simulink model "Backhoe_Arm"  (R2020a)
settings: Solver=ode23t  StartTime=0.0  StopTime=60  RelTol=1e-3  EnableMultiTasking=on
PostLoadFcn:
  | warning off simscape:compiler:sli:init:SolverNotRecommended
  | 
  | warning off sm:sli:visualization:UnsupportedSimMode
  | warning off sm:sli:setup:compile:LocalSolverNotSupported
  | warning off sm:compiler:state:UnsatisfiedDesiredTarget
  | 
  | warning off xPCTarget:sampleTime:sampleTimeInvariance
  | warning off Simulink:blocks:MatchingFromNotFound
model workspace (MAT data in the model file):
  cylinderGray = [0.6 0.6 0.6]
  darkOrange = [0.8 0.5 0]
  glassBlue = [0.2 0.2 1]
  gray = [0.3 0.3 0.3]
  orange = [0.8 0.65 0]
  pistonGray = [0.4 0.4 0.4]
  rhoGlass = 2500
  rhoRubber = 1500
  rhoSteel = 7800
  tireBlack = [0.1 0.1 0.1]
  wheelGray = [0.6 0.6 0.6]
  yellow = [0.8 0.8 0]
undefined symbols (not defined in the file or in its folder): BH_Param, sigbuilder_block, X, Y, Z
libraries: sm_lib x98, fl_lib x31, Backhoe_Lib x28, nesl_utility x22, sh_lib x9, slrtlib x1
(part 1 of 4)
CloseFcn:
  | try,close(h1_Backhoe_Arm),end
  | clear h1_Backhoe_Arm
  | try,close(h2_Backhoe_Arm),end
  | clear h2_Backhoe_Arm
  | 
  | clear simlog_Backhoe_Arm
  | clear logsout_Backhoe_Arm
Description:
  | Backhoe Arm
  | 
  | Copyright 2014-2020 The MathWorks, Inc.
settings Model: ExtModeTrigDuration=2500  Creator=smiller  LastModifiedBy=smiller
settings DataIOCC: MaxDataPoints=10000  SaveFormat=Array  ReturnWorkspaceOutputs=off  SignalLoggingName=logsout_Backhoe_Arm
settings OptimizationCC: BlockReduction=off  OptimizeBlockIOStorage=off  BufferReuse=off  GlobalBufferReuse=off  ExpressionFolding=off  ExpressionDepthLimit=2147483647  LocalBlockOutputs=off  LifeSpan=inf  OptimizeDataStoreBuffers=off  BusAssignmentInplaceUpdate=off
settings DebuggingCC: UnderspecifiedInitializationDetection=Classic  MergeDetectMultiDrivingBlocksExec=none  MultiTaskDSMMsg=warning  MultiTaskCondExecSysMsg=none  AllowSymbolicDim=off  StateNameClashWarn=warning  PregeneratedLibrarySubsystemCodeDiagnostic=none  SFUnexpectedBacktrackingDiag=warning  SFNoUnconditionalDefaultTransitionDiag=warning  SFExecutionAtInitializationDiag=none  ArithmeticOperatorsInVariantConditions=warning
settings HardwareCC: ProdBitPerPointer=32  ProdBitPerSizeT=32  ProdBitPerPtrDiffT=32  ProdLargestAtomicFloat=None  ProdWordSize=32  ProdLongLongMode=on  ProdHWDeviceType=Generic->32-bit x86 compatible
settings ModelReferenceCC: PropagateSignalLabelsOutOfModel=off
settings SFSimCC: SimUseLocalCustomCode=off  CustomCodeUndefinedFunction=UseInterfaceOnly
settings RTWCC: Description=Simulink Real-Time  SystemTargetFile=slrt.tlc  TemplateMakefile=slrt_default_tmf  RTWUseLocalCustomCode=off  CodeExecutionProfiling=on  RTWCompilerOptimization=on
settings CodeAppCC: StateflowObjectComments=on
settings SimulinkRealTimeCC: RL32LogBufSizeModifier=300000
settings ConfigComp: CovMetricSettings=dw  CovHtmlReporting=on  CovSaveCumulativeToWorkspaceVar=on  CovSaveSingleToWorkspaceVar=on  CovExternalEMLEnable=off  CovSFcnEnable=off
settings SimscapeCC: ExplicitSolverDiagnosticOptions=none  SimscapeNormalizeSystem=off  SimscapeLogType=all  SimscapeLogSimulationStatistics=on  SimscapeLogName=simlog_Backhoe_Arm  SimscapeLogDataHistory=150000
settings ConfigurationSet: Description=SimMechanics 2G
settings ExplorerConfigSet: InternalSimMechanicsExplorerSettings="<ExplorerConfiguration><canonicalview>default</canonicalview><AnimationSetting><BasePlaybackSpeed>1.0</BasePlaybackSpeed><PlaybackSpeedFactor>1.0</PlaybackSpeedFactor></AnimationSetting><TilePanel><TileInfo><Tiles Columns=\"1\" Count=\"1\" Rows=\"1\"><Column Weight=\"1\"/><Row Weight=\"1\"/><Tile Height=\"1\" Width=\"1\" X=\"0\" Y=\"0\"/></Tiles></TileInfo><SceneInfo><SceneViewer><BGColor><R>1</R><G>1</G><B>1</B></BGColor><Camera><DoPerspective>off</DoPerspective><Position><X>16.2117166228468328</X><Y>-13.0612993780048647</Y><Z>8.35403361976682568</Z></Position><Center><X>-0.886183199059584648</X><Y>-6.57974503836197222</Y><Z>3.30771103067373451</Z></Center><Up><X>-0.262324217563679185</X><Y>0.057951672533943753</Y><Z>0.963238085070416306</Z></Up><ViewLimDist>1</ViewLimDist><YLim>5.09128224849700928</YLim><XLim>8.0878249386863228</XLim></Camera></SceneViewer></SceneInfo></TilePanel><MechEditorPanel><Cameras/><GfxPanelCameraMap/><VideoCreator><PlaybackSpeedRatio>1.0</PlaybackSpeedRatio><FrameRate>30</FrameRate><VideoFormat>Motion JPEG AVI</VideoFormat><FrameSize>auto</FrameSize></VideoCreator></MechEditorPanel></ExplorerConfiguration>"

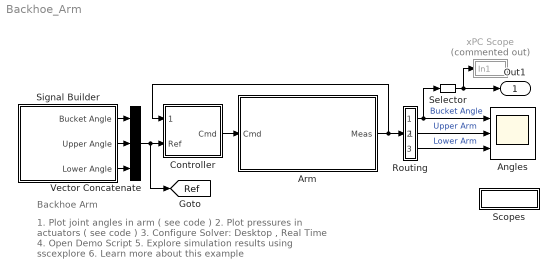
== system Backhoe_Arm ==
  note: 1. Plot joint angles in arm ( see code )
      | 2. Plot pressures in actuators ( see code )
      | 3. Configure Solver: Desktop , Real Time
      | 4. Open Demo Script
      | 5. Explore simulation results using sscexplore
      | 6. Learn more about this example
  note: Backhoe Arm
  Angles : Scope  NumInputPorts=3
  Arm : Subsystem  Tag=PublishSubsystem
      mask Display:
      | image('Backhoe_Arm_IMAGE.jpg');
      | port_label('input',1,'Cmd');
      | port_label('Output',1,'Meas');
  Controller : Subsystem
  Routing : Subsystem
  Scopes : Subsystem
  Selector : Selector  InputPortWidth=2  IndexOptions=Index vector (dialog)  Indices=[1]  OutputSizes=1
  Signal Builder : Subsystem  Tag=STV Subsys  LoadFcn=sigbuilder_block('load');  StartFcn=sigbuilder_block('start');  StopFcn=sigbuilder_block('stop');  ClipboardFcn=sigbuilder_block('clipboard');  mask(Sigbuilder block){tuvar=[0:10]}
      mask help: Simulink:masks:SigbuilderBlock_MD
      mask init:
      | if ~strcmp(get_param(bdroot(gcbh),'SimulationStatus'),'stopped') tuvar = sigbuilder_block('maskInit'); end
      settings: CopyFcn=sigbuilder_block('copy');  DeleteFcn=sigbuilder_block('delete');  ModelCloseFcn=sigbuilder_block('modelClose');  PreSaveFcn=sigbuilder_block('preSave');  PauseFcn=sigbuilder_block('pause');  ContinueFcn=sigbuilder_block('continue');  NameChangeFcn=sigbuilder_block('namechange');  OpenFcn=sigbuilder_block('open',[5.58621 8.06897 624.414 412.759 ]);  CloseFcn=sigbuilder_block('close');
      mask Display: plot(0, 0, 100, 100,[2, 2, 32, 32, 2], [68, 8, 8, 68, 68],[32, 2], [38, 38], [32, 19, 2],[53, 60, 44], [32, 17, 17, 2],[16, 16, 31, 31]);txt = getActiveGroup(gcbh);text(2, 100, txt,'verticalAlignment', 'top');
  Vector Concatenate : Concatenate  NumInputs=3
  xPC Scope : Subsystem  Commented=on
      mask Display: disp('SLRT')
  Out1 : Outport  VectorParamsAs1DForOutWhenUnconnected=off
  tag scope: Ref=global
  wires:
  Signal Builder/2(Upper Angle) -> Vector Concatenate/2
  Signal Builder/1(Bucket Angle) -> Vector Concatenate/1
  Signal Builder/3(Lower Angle) -> Vector Concatenate/3
  Vector Concatenate/1 -> [Ref], Controller/2(Ref)
  Arm/1(Meas) -> Controller/1(Meas), Routing/1(Meas)
  Controller/1(Cmd) -> Arm/1(Cmd)
  Routing/2(UArm) -> Angles/2  "Upper Arm"
  Routing/3(LArm) -> Angles/3  "Lower Arm"
  Routing/1(Bucket) -> Selector/1, Angles/1  "Bucket Angle"
  Selector/1 -> xPC Scope/1(In1), Out1/1

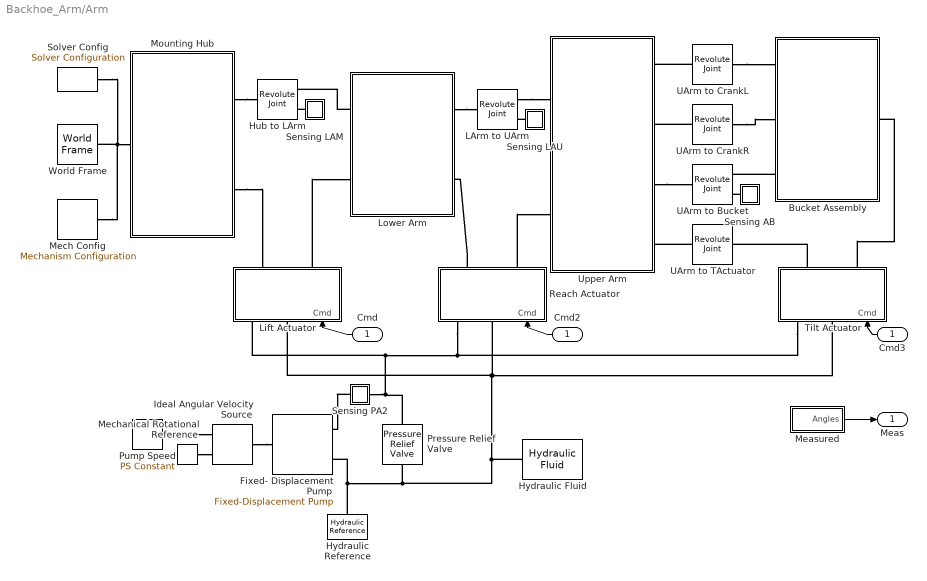
== system Backhoe_Arm/Arm ==
  Cmd : Inport
  Bucket Assembly : Subsystem
      mask Display: image('Backhoe_Arm_Bucket_Asy_IMAGE.jpg');
  Cmd2 : InportShadow
  Cmd3 : InportShadow
  Fixed- Displacement Pump : sh_lib/Pumps and Motors/Fixed-Displacement Pump  D=BH_Param.Hydraulic.Pump.Displacement m^3/rad  loss_spec=1  w_nominal=BH_Param.Hydraulic.Pump.Nominal_Ang_Vel rad/s  pr_nominal=BH_Param.Hydraulic.Pump.Nominal_Pressure Pa  visc_nominal=BH_Param.Hydraulic.Pump.Nominal_Kin_Visc cSt  dens_nominal=900 kg/m^3  efficiency_vol=BH_Param.Hydraulic.Pump.Vol_Eff  no_load_torque=0 N*m  torque_pressure_coeff=1*(BH_Param.Hydraulic.Pump.Displacement)*((BH_Param.Hydraulic.Pump.Vol_Eff)/(BH_Param.Hydraulic.Pump.Total_Eff)-1 ) N*m/Pa  p_diff_eff_TLU=[100000.0, 1000000.0, 2000000.0] Pa  omega_eff_TLU=[25.0, 50.0, 100.0, 200.0, 300.0, 400.0] rad/s  vol_eff_TLU=[0.816, 0.908, 0.954, 0.977, 0.981, 0.984; 0.325, 0.663, 0.831, 0.916, 0.925, 0.946; 0.137, 0.568, 0.78, 0.892, 0.893, 0.91]  mech_eff_TLU=[0.996, 0.996, 0.996, 0.996, 0.996, 0.996; 0.988, 0.989, 0.989, 0.989, 0.989, 0.99; 0.981, 0.981, 0.982, 0.982, 0.983, 0.984]  p_diff_loss_TLU=[100000.0, 1000000.0, 2000000.0] Pa  omega_loss_TLU=[25.0, 50.0, 100.0, 200.0, 300.0, 400.0] rad/s  vol_loss_TLU=[0.023, 0.023, 0.023, 0.023, 0.0285, 0.032; 0.0844, 0.0842, 0.0845, 0.084, 0.1125, 0.108; 0.1079, 0.108, 0.11, 0.108, 0.1605, 0.18] * 1e-3 m^3/s  mech_loss_TLU=[0.002, 0.002, 0.002, 0.002, 0.002, 0.002; 0.0607, 0.0556, 0.0556, 0.0556, 0.0556, 0.0505; 0.1937, 0.1937, 0.1833, 0.1833, 0.1729, 0.1626] N*m  pressure_threshold=1e5 Pa  omega_threshold=10 rad/s  quadrant_check=0  pressure_check=0  min_valid_pressure=0 Pa  vol_eff_min=1e-3  vol_eff_max=1  mech_eff_min=1e-3  mech_eff_max=1
      settings: SourceProductBaseCode=SH  InternalSimscapePortConfiguration="{\"Bottom\":[],\"Left\":[{\"id\":\"S\",\"label\":\"S\",\"type\":\"foundation.mechanical.rotational.rotational\"}],\"Right\":[{\"id\":\"P\",\"label\":\"P\",\"type\":\"foundation.hydraulic.hydraulic\"},{\"id\":\"T\",\"label\":\"T\",\"type\":\"foundation.hydraulic.hydraulic\"}],\"Top\":[]}"
  Hub to LArm : sm_lib/Joints/Revolute Joint  JointMode=Normal  SenseConstraintForce=off  SenseConstraintForceX=off  SenseConstraintForceY=off  SenseConstraintForceZ=off  SenseConstraintTorque=off  SenseConstraintTorqueX=off  SenseConstraintTorqueY=off  SenseConstraintTorqueZ=off  SenseTotalForce=off  SenseTotalForceX=off  SenseTotalForceY=off  SenseTotalForceZ=off  SenseTotalTorque=off  SenseTotalTorqueX=off  SenseTotalTorqueY=off  SenseTotalTorqueZ=off  CompositeWrenchDir=FollowerOnBase  CompositeWrenchFrame=BaseFrame  EquilibriumPosition=0  EquilibriumPositionUnits=deg  SpringStiffness=0  SpringStiffnessUnits=N*m/deg  DampingCoefficient=0  DampingCoefficientUnits=N*m/(deg/s)  TorqueActuationMode=NoTorque  MotionActuationMode=ComputedMotion  SensePosition=on  SenseVelocity=off  SenseAcceleration=off  SenseTorqueForce=off  SenseLowerLimitTorqueForce=off  SenseUpperLimitTorqueForce=off  LowerLimitSpecify=off  LowerLimitBound=-90  LowerLimitBoundUnits=deg  LowerLimitStiffness=1e4  LowerLimitStiffnessUnits=N*m/deg  LowerLimitDamping=10  LowerLimitDampingUnits=N*m/(deg/s)  LowerLimitTransitionRegionWidth=0.1  LowerLimitTransitionRegionWidthUnits=deg  UpperLimitSpecify=off  UpperLimitBound=90  UpperLimitBoundUnits=deg  UpperLimitStiffness=1e4  UpperLimitStiffnessUnits=N*m/deg  UpperLimitDamping=10  UpperLimitDampingUnits=N*m/(deg/s)  UpperLimitTransitionRegionWidth=0.1  UpperLimitTransitionRegionWidthUnits=deg  PositionTargetSpecify=on  PositionTargetPriority=High  PositionTargetValue=-60  PositionTargetValueUnits=deg  VelocityTargetSpecify=off  VelocityTargetPriority=High  VelocityTargetValue=0  VelocityTargetValueUnits=deg/s
  Hydraulic Reference : fl_lib/Hydraulic/Hydraulic Elements/Hydraulic Reference
  Hydraulic Fluid : sh_lib/Hydraulic Utilities/Hydraulic Fluid  DataSource=1  SelFluid=9  SysTemp=50  TrapAir=0.004  ViscDerFactor=1  range_error=2
  Ideal Angular Velocity Source : fl_lib/Mechanical/Mechanical Sources/Ideal Angular Velocity Source
  LArm to UArm : sm_lib/Joints/Revolute Joint  JointMode=Normal  SenseConstraintForce=off  SenseConstraintForceX=off  SenseConstraintForceY=off  SenseConstraintForceZ=off  SenseConstraintTorque=off  SenseConstraintTorqueX=off  SenseConstraintTorqueY=off  SenseConstraintTorqueZ=off  SenseTotalForce=off  SenseTotalForceX=off  SenseTotalForceY=off  SenseTotalForceZ=off  SenseTotalTorque=off  SenseTotalTorqueX=off  SenseTotalTorqueY=off  SenseTotalTorqueZ=off  CompositeWrenchDir=FollowerOnBase  CompositeWrenchFrame=BaseFrame  EquilibriumPosition=0  EquilibriumPositionUnits=deg  SpringStiffness=0  SpringStiffnessUnits=N*m/deg  DampingCoefficient=0  DampingCoefficientUnits=N*m/(deg/s)  TorqueActuationMode=NoTorque  MotionActuationMode=ComputedMotion  SensePosition=on  SenseVelocity=off  SenseAcceleration=off  SenseTorqueForce=off  SenseLowerLimitTorqueForce=off  SenseUpperLimitTorqueForce=off  LowerLimitSpecify=off  LowerLimitBound=-90  LowerLimitBoundUnits=deg  LowerLimitStiffness=1e4  LowerLimitStiffnessUnits=N*m/deg  LowerLimitDamping=10  LowerLimitDampingUnits=N*m/(deg/s)  LowerLimitTransitionRegionWidth=0.1  LowerLimitTransitionRegionWidthUnits=deg  UpperLimitSpecify=off  UpperLimitBound=90  UpperLimitBoundUnits=deg  UpperLimitStiffness=1e4  UpperLimitStiffnessUnits=N*m/deg  UpperLimitDamping=10  UpperLimitDampingUnits=N*m/(deg/s)  UpperLimitTransitionRegionWidth=0.1  UpperLimitTransitionRegionWidthUnits=deg  PositionTargetSpecify=on  PositionTargetPriority=High  PositionTargetValue=50  PositionTargetValueUnits=deg  VelocityTargetSpecify=off  VelocityTargetPriority=High  VelocityTargetValue=0  VelocityTargetValueUnits=deg/s
  Lift Actuator : Subsystem  Tag=PublishSubsystem  mask(Hydraulic Actuator){Lcyl=BH_Param.Lift_Actuator.Cyl_Dims.Lcyl, Rcyl=BH_Param.Lift_Actuator.Cyl_Dims.Rcyl, Lbase=BH_Param.Lift_Actuator.Cyl_Dims.Lbase, Wbase=BH_Param.Lift_Actuator.Cyl_Dims.Wbase, Rbp=BH_Param.Lift_Actuator.Cyl_Dims.Rbp, Lbp=BH_Param.Lift_Actuator.Cyl_Dims.Lbp, Lpist=BH_Param.Lift_Actuator.Piston_Dims.Lpist, Rpist=BH_Param.Lift_Actuator.Piston_Dims.Rpist, Whead=BH_Param.Lift_Actuator.Piston_Dims.Whead, Lhead=BH_Param.Lift_Actuator.Piston_Dims.Lhead, Rhp=BH_Param.Lift_Actuator.Piston_Dims.Rhp, Lhp=BH_Param.Lift_Actuator.Piston_Dims.Lhp, hydr_area=BH_Param.Lift_Actuator.Cylinder.Area_A, hydr_stroke=BH_Param.Lift_Actuator.Cylinder.Stroke, hydr_deadvol=BH_Param.Lift_Actuator.Cylinder.DeadVol_A, hydr_x0=BH_Param.Lift_Actuator.Cylinder.x0, hydr_PA0=BH_Param.Lift_Actuator.Cylinder.PA0, hydr_PB0=BH_Param.Lift_Actuator.Cylinder.PB0, hydr_valve_max_area=BH_Param.Lift_Actuator.Valve.Max_Area, hydr_valve_max_opening=BH_Param.Lift_Actuator.Valve.Max_Opening, friction_breakaway=BH_Param.Lift_Actuator.Friction.Breakaway, friction_coulomb=BH_Param.Lift_Actuator.Friction.Coulomb, friction_viscous=BH_Param.Lift_Actuator.Friction.Viscous, circlePoints=25, cylColor=BH_Param.Colors.cylinderGray, rhoCyl=BH_Param.Densities.rhoSteel, pistColor=BH_Param.Colors.pistonGray, rhoPist=BH_Param.Densities.rhoSteel, connColor=BH_Param.Colors.gray, rhoConn=BH_Param.Densities.rhoSteel}
      mask prompts: Lcyl "Lcyl [m]"; Rcyl "Rcyl [m]"; Lbase "Lbase [m]"; Wbase "Wbase [m]"; Rbp "Rbp [m]"; Lbp "Lbp [m]"; Lpist "Lpist [m]"; Rpist "Rpist [m]"; Whead "Whead [m]"; Lhead "Lhead [m]"; Rhp "Rhp [m]"; Lhp "Lhp [m]"; hydr_area "Piston Area [m^3]"; hydr_stroke "Piston Stroke [m]"; hydr_deadvol "Dead Volume [m^3]"; hydr_x0 "Initial Position [m]"; hydr_PA0 "Initial Pressure, Chamber A [Pa]"; hydr_PB0 "Initial Pressure, Chamber B [Pa]"; hydr_valve_max_area "Valve Max Area [mm^2]"; hydr_valve_max_opening "Valve Max Opening [m]"; friction_breakaway "Breakaway Friction Force [N]"; friction_coulomb "Coulomb Friction Force [N]"; friction_viscous "Viscous Friction Coefficient [N/(m/2)]"; circlePoints "Circle Mesh Resolution"; cylColor "Cylinder Color"; rhoCyl "Cylinder Density [kg/m^3]"; pistColor "Piston Color"; rhoPist "Piston Density [kg/m^3]"; connColor "Connector Color"; rhoConn "Connector Density [kg/m^3]"
      mask help:
      | Consists of the backhoe hydraulic actuator assembly.
      |
      | Zero piston displacement corresponds to the piston and cylinder centers of mass in the same position. Positive piston displacement is outward motion, and negative piston displacement is inward motion.
      |
      | Attachment points are:
      | C: Center of the Cylinder base bracket hole.
      | H: Center of the Piston Head bracket hole.
      | Both attachment points are configured for Revolute joints.
      |
      | The Simulink Signal input port supplies a Pressure value P (in Pa) to a Simscape hydraulic network.
      |
      | Click on Help to view a schematic of the hydraulic actuator, its configurable dimension parameters and attachment points (in red).
      mask init:
      | % Hollow Cylinder cross-section
      | cylSection = [];
      | 
      | for i = 0:2*circlePoints
      |     angle = (i/circlePoints)*pi;
      |     cylSection = [cylSection; Rcyl*cos(angle) Rcyl*sin(angle)];
      | end
      | 
      | for i = 0:2*circlePoints
      |     angle = -(i/circlePoints)*pi;
      |     cylSection = [cylSection; Rpist*cos(angle) Rpist*sin(angle)];
      | end
      mask Help: web('Backhoe_Actuator.html');
      mask DialogControl ParameterTabVar0 Prompt: Cylinder
      mask DialogControl ParameterTabVar01 Prompt: Piston
      mask DialogControl ParameterTabVar012 Prompt: Hydraulic
      mask DialogControl ParameterTabVar0123 Prompt: Friction
      mask DialogControl ParameterTabVar01234 Prompt: Other
      mask Display: image('Backhoe_Arm_Actuator_IMAGE.jpg');
  "Lower Arm " : Subsystem
      mask Display: image('Backhoe_Arm_Lower_IMAGE.jpg');
  Measured : Subsystem
  Mech Config : sm_lib/Utilities/Mechanism Configuration  UniformGravity=Constant  GravityVector=[0 0 -9.81]  GravityUnits=m/s^2  LinearizationDelta=0.001
  Mechanical Rotational Reference : fl_lib/Mechanical/Rotational Elements/Mechanical Rotational Reference
  Mounting Hub : Subsystem  mask(Mounting Hub){Hleft=1, Hright=2, Ltop=0.75, Lbottom=1.5, Tplate=0.3, Dplates=1.2, plateFillet=0.25, numPoints=15, L1=0.75, H1=0.25, RH1=0.075, L2=0.75, H2=1.75, RH2=0.075, L3=0.5, H3=0.5, Larm=0.8, Warm=0.5, Tarm=0.5, Tab=0.1, RH3=0.075, Dbracket=1.1, Lbracket=1.2, Wbracket=1.2, Tbracket=2, Hbracket=1, Rhole=0.1, Hhole=0.5, hubColor=orange, rho=rhoSteel}
      mask prompts: Hleft "Hleft [m]"; Hright "Hright [m]"; Ltop "Ltop [m]"; Lbottom "Lbottom [m]"; Tplate "Tplate [m]"; Dplates "Dplates [m]"; plateFillet "Plate Fillet Radius [m]"; numPoints "Fillet Point Resolution"; L1 "L1 [m]"; H1 "H1 [m]"; RH1 "RH1 [m]"; L2 "L2 [m]"; H2 "H2 [m]"; RH2 "RH2 [m]"; L3 "L3 [m]"; H3 "H3 [m]"; Larm "Larm [m]"; Warm "Warm [m]"; Tarm "Tarm [m]"; Tab "Tab [m]"; RH3 "RH3 [m]"; Dbracket "Dbracket [m]"; Lbracket "Lbracket [m]"; Wbracket "Wbracket [m]"; Tbracket "Tbracket [m]"; Hbracket "Hbracket [m]"; Rhole "Rhole [m]"; Hhole "Hhole [m]"; hubColor "Hub Color"; rho "Density [kg/m^3]"
      mask help:
      | Consists of the backhoe mounting hub assembly.
      |
      | This assembly connects to the Backhoe Arm assembly on the front end, and to the Mounting Base assembly on the rear and side.
      |
      | Attachment points are:
      | LH: Left base hydraulic actuator (piston Head).
      | RH: Right base hydraulic actuator (piston Head).
      | LC: Lower arm hydraulic actuator (Cylinder base).
      | LA: Lower Arm joint.
      | MB: Mounting Base joint.
      | All attachments are configured for Revolute Joints.
      |
      | Click on Help to view a schematic of the bracket, its configurable dimension parameters and attachment points (in red).
      mask init:
      | plateSection = [0              0     ; ...
      |                 Lbottom        0     ; ...
      |                 Lbottom        Hright; ...
      |                 (Lbottom-Ltop) Hright; ...
      |                 0              Hleft];
      | plateSection = Extr_Data_Round_Corners(plateSection,1:5,0.1,15);
      mask Help: web('Backhoe_Mountinghub.html');
      mask DialogControl ParameterTabVar0 Prompt: Plate
      mask DialogControl ParameterTabVar01 Prompt: Pins
      mask DialogControl ParameterTabVar012 Prompt: Attachment Arms
      mask DialogControl ParameterTabVar0123 Prompt: Bracket
      mask DialogControl ParameterTabVar01234 Prompt: Material Properties
      mask Display: image('Backhoe_Arm_Base_IMAGE.jpg');
  Pressure Relief Valve : sh_lib/Valves/Pressure Control Valves/Pressure Relief Valve  valve_area_spec=1  p_diff_TLU=[30.15e5 : 15e3 : 31.35e5] Pa  area_TLU=[1 : 1 : 9] .* 1e-5 m^2  area_max=BH_Param.Hydraulic.PRV.Max_Area m^2  pres_set=BH_Param.Hydraulic.PRV.Pressure_Set Pa  reg_range=BH_Param.Hydraulic.PRV.Pressure_Rng Pa  C_d=BH_Param.Hydraulic.PRV.Flow_Disch_Coeff  A_leak=BH_Param.Hydraulic.PRV.Leakage_Area m^2  lam_spec=2  B_lam=0.999  Re_cr=BH_Param.Hydraulic.PRV.Re_Critical  dynamic=0  tau=0.1 s  area_init=1e-12 m^2
      settings: SourceProductBaseCode=SH  InternalSimscapePortConfiguration="{\"Bottom\":[],\"Left\":[{\"id\":\"A\",\"label\":\"A\",\"type\":\"foundation.hydraulic.hydraulic\"}],\"Right\":[{\"id\":\"B\",\"label\":\"B\",\"type\":\"foundation.hydraulic.hydraulic\"}],\"Top\":[]}"
  Pump Speed : fl_lib/Physical Signals/Sources/PS Constant  constant=BH_Param.Hydraulic.Pump.Speed
  Reach Actuator : Subsystem  mask(Hydraulic Actuator){Lcyl=BH_Param.Reach_Actuator.Cyl_Dims.Lcyl, Rcyl=BH_Param.Reach_Actuator.Cyl_Dims.Rcyl, Lbase=BH_Param.Reach_Actuator.Cyl_Dims.Lbase, Wbase=BH_Param.Reach_Actuator.Cyl_Dims.Wbase, Rbp=BH_Param.Reach_Actuator.Cyl_Dims.Rbp, Lbp=BH_Param.Reach_Actuator.Cyl_Dims.Lbp, Lpist=BH_Param.Reach_Actuator.Piston_Dims.Lpist, Rpist=BH_Param.Reach_Actuator.Piston_Dims.Rpist, Whead=BH_Param.Reach_Actuator.Piston_Dims.Whead, Lhead=BH_Param.Reach_Actuator.Piston_Dims.Lhead, Rhp=BH_Param.Reach_Actuator.Piston_Dims.Rhp, Lhp=BH_Param.Reach_Actuator.Piston_Dims.Lhp, hydr_area=BH_Param.Reach_Actuator.Cylinder.Area_A, hydr_stroke=BH_Param.Reach_Actuator.Cylinder.Stroke, hydr_deadvol=BH_Param.Reach_Actuator.Cylinder.DeadVol_A, hydr_x0=BH_Param.Reach_Actuator.Cylinder.x0, hydr_PA0=BH_Param.Reach_Actuator.Cylinder.PA0, hydr_PB0=BH_Param.Reach_Actuator.Cylinder.PB0, hydr_valve_max_area=BH_Param.Reach_Actuator.Valve.Max_Area, hydr_valve_max_opening=BH_Param.Reach_Actuator.Valve.Max_Opening, friction_breakaway=BH_Param.Reach_Actuator.Friction.Breakaway, friction_coulomb=BH_Param.Reach_Actuator.Friction.Coulomb, friction_viscous=BH_Param.Reach_Actuator.Friction.Viscous, circlePoints=25, cylColor=BH_Param.Colors.cylinderGray, rhoCyl=BH_Param.Densities.rhoSteel, pistColor=BH_Param.Colors.pistonGray, rhoPist=BH_Param.Densities.rhoSteel, connColor=BH_Param.Colors.gray, rhoConn=BH_Param.Densities.rhoSteel}
      mask prompts: Lcyl "Lcyl [m]"; Rcyl "Rcyl [m]"; Lbase "Lbase [m]"; Wbase "Wbase [m]"; Rbp "Rbp [m]"; Lbp "Lbp [m]"; Lpist "Lpist [m]"; Rpist "Rpist [m]"; Whead "Whead [m]"; Lhead "Lhead [m]"; Rhp "Rhp [m]"; Lhp "Lhp [m]"; hydr_area "Piston Area [m^3]"; hydr_stroke "Piston Stroke [m]"; hydr_deadvol "Dead Volume [m^3]"; hydr_x0 "Initial Position [m]"; hydr_PA0 "Initial Pressure, Chamber A [Pa]"; hydr_PB0 "Initial Pressure, Chamber B [Pa]"; hydr_valve_max_area "Valve Max Area [mm^2]"; hydr_valve_max_opening "Valve Max Opening [m]"; friction_breakaway "Breakaway Friction Force [N]"; friction_coulomb "Coulomb Friction Force [N]"; friction_viscous "Viscous Friction Coefficient [N/(m/2)]"; circlePoints "Circle Mesh Resolution"; cylColor "Cylinder Color"; rhoCyl "Cylinder Density [kg/m^3]"; pistColor "Piston Color"; rhoPist "Piston Density [kg/m^3]"; connColor "Connector Color"; rhoConn "Connector Density [kg/m^3]"
      mask help:
      | Consists of the backhoe hydraulic actuator assembly.
      |
      | Zero piston displacement corresponds to the piston and cylinder centers of mass in the same position. Positive piston displacement is outward motion, and negative piston displacement is inward motion.
      |
      | Attachment points are:
      | C: Center of the Cylinder base bracket hole.
      | H: Center of the Piston Head bracket hole.
      | Both attachment points are configured for Revolute joints.
      |
      | The Simulink Signal input port supplies a Pressure value P (in Pa) to a Simscape hydraulic network.
      |
      | Click on Help to view a schematic of the hydraulic actuator, its configurable dimension parameters and attachment points (in red).
      mask init: same as Backhoe_Arm/Arm/Lift Actuator
      mask Help: web('Backhoe_Actuator.html');
      mask DialogControl ParameterTabVar0 Prompt: Cylinder
      mask DialogControl ParameterTabVar01 Prompt: Piston
      mask DialogControl ParameterTabVar012 Prompt: Hydraulic
      mask DialogControl ParameterTabVar0123 Prompt: Friction
      mask DialogControl ParameterTabVar01234 Prompt: Other
      mask Display: image('Backhoe_Arm_Actuator_IMAGE.jpg');
  Sensing AB : Subsystem
      mask Display: disp('S')
  Sensing LAM : Subsystem
      mask Display: disp('S')
  Sensing LAU : Subsystem
      mask Display: disp('S')
  Sensing PA2 : Subsystem
      mask Display: disp('S')
  Solver Config : nesl_utility/Solver Configuration  PhysicalDomain=network_engine_domain  SubClassName=solver  LeftPortType=input  RightPortType=generic  Tones=[]  Harmonics=[]  SimulateNoise=off  Profile=off  UseLocalSampling=off  EnableSwitchedLinearOptims=on  FrequencyDomain=off  UseCCode=off  RelTol=0.001  AbsTol=1e-06  MinStep=1e-09  ToWorkspace=off  RevertToSquareIcSolve=off  NumHomotopyIterations=100  PhasorMode=off  PhasorModeNumHarmonics=1  DoDC=off  ResidualTolerance=1e-9  UseLocalSolver=off  LocalSolverChoice=NE_BACKWARD_EULER_ADVANCER  LocalSolverSampleTime=0.0004  DoFixedCost=off  MaxNonlinIter=2  MaxModeIter=2  LinearAlgebra=Sparse  EquationFormulation=NE_TIME_EF  DelaysMemoryBudget=1024  AutomaticFiltering=on  FilteringTimeConstant=0.001  PartitionStorageMethod=AS_NEEDED  PartitionMemoryBudget=1024  PartitionMethod=FAST
  Tilt Actuator : Subsystem  mask(Hydraulic Actuator){Lcyl=BH_Param.Tilt_Actuator.Cyl_Dims.Lcyl, Rcyl=BH_Param.Tilt_Actuator.Cyl_Dims.Rcyl, Lbase=BH_Param.Tilt_Actuator.Cyl_Dims.Lbase, Wbase=BH_Param.Tilt_Actuator.Cyl_Dims.Wbase, Rbp=BH_Param.Tilt_Actuator.Cyl_Dims.Rbp, Lbp=BH_Param.Tilt_Actuator.Cyl_Dims.Lbp, Lpist=BH_Param.Tilt_Actuator.Piston_Dims.Lpist, Rpist=BH_Param.Tilt_Actuator.Piston_Dims.Rpist, Whead=BH_Param.Tilt_Actuator.Piston_Dims.Whead, Lhead=BH_Param.Tilt_Actuator.Piston_Dims.Lhead, Rhp=BH_Param.Tilt_Actuator.Piston_Dims.Rhp, Lhp=BH_Param.Tilt_Actuator.Piston_Dims.Lhp, hydr_area=BH_Param.Tilt_Actuator.Cylinder.Area_A, hydr_stroke=BH_Param.Tilt_Actuator.Cylinder.Stroke, hydr_deadvol=BH_Param.Tilt_Actuator.Cylinder.DeadVol_A, hydr_x0=BH_Param.Tilt_Actuator.Cylinder.x0, hydr_PA0=BH_Param.Tilt_Actuator.Cylinder.PA0, hydr_PB0=BH_Param.Tilt_Actuator.Cylinder.PB0, hydr_valve_max_area=BH_Param.Tilt_Actuator.Valve.Max_Area, hydr_valve_max_opening=BH_Param.Tilt_Actuator.Valve.Max_Opening, friction_breakaway=BH_Param.Tilt_Actuator.Friction.Breakaway, friction_coulomb=BH_Param.Tilt_Actuator.Friction.Coulomb, friction_viscous=BH_Param.Tilt_Actuator.Friction.Viscous, circlePoints=25, cylColor=BH_Param.Colors.cylinderGray, rhoCyl=BH_Param.Densities.rhoSteel, pistColor=BH_Param.Colors.pistonGray, rhoPist=BH_Param.Densities.rhoSteel, connColor=BH_Param.Colors.gray, rhoConn=BH_Param.Densities.rhoSteel}
      mask prompts: Lcyl "Lcyl [m]"; Rcyl "Rcyl [m]"; Lbase "Lbase [m]"; Wbase "Wbase [m]"; Rbp "Rbp [m]"; Lbp "Lbp [m]"; Lpist "Lpist [m]"; Rpist "Rpist [m]"; Whead "Whead [m]"; Lhead "Lhead [m]"; Rhp "Rhp [m]"; Lhp "Lhp [m]"; hydr_area "Piston Area [m^3]"; hydr_stroke "Piston Stroke [m]"; hydr_deadvol "Dead Volume [m^3]"; hydr_x0 "Initial Position [m]"; hydr_PA0 "Initial Pressure, Chamber A [Pa]"; hydr_PB0 "Initial Pressure, Chamber B [Pa]"; hydr_valve_max_area "Valve Max Area [mm^2]"; hydr_valve_max_opening "Valve Max Opening [m]"; friction_breakaway "Breakaway Friction Force [N]"; friction_coulomb "Coulomb Friction Force [N]"; friction_viscous "Viscous Friction Coefficient [N/(m/2)]"; circlePoints "Circle Mesh Resolution"; cylColor "Cylinder Color"; rhoCyl "Cylinder Density [kg/m^3]"; pistColor "Piston Color"; rhoPist "Piston Density [kg/m^3]"; connColor "Connector Color"; rhoConn "Connector Density [kg/m^3]"
      mask help:
      | Consists of the backhoe hydraulic actuator assembly.
      |
      | Zero piston displacement corresponds to the piston and cylinder centers of mass in the same position. Positive piston displacement is outward motion, and negative piston displacement is inward motion.
      |
      | Attachment points are:
      | C: Center of the Cylinder base bracket hole.
      | H: Center of the Piston Head bracket hole.
      | Both attachment points are configured for Revolute joints.
      |
      | The Simulink Signal input port supplies a Pressure value P (in Pa) to a Simscape hydraulic network.
      |
      | Click on Help to view a schematic of the hydraulic actuator, its configurable dimension parameters and attachment points (in red).
      mask init: same as Backhoe_Arm/Arm/Lift Actuator
      mask Help: web('Backhoe_Actuator.html');
      mask DialogControl ParameterTabVar0 Prompt: Cylinder
      mask DialogControl ParameterTabVar01 Prompt: Piston
      mask DialogControl ParameterTabVar012 Prompt: Hydraulic
      mask DialogControl ParameterTabVar0123 Prompt: Friction
      mask DialogControl ParameterTabVar01234 Prompt: Other
      mask Display: image('Backhoe_Arm_Actuator_IMAGE.jpg');
  UArm to Bucket : sm_lib/Joints/Revolute Joint  JointMode=Normal  SenseConstraintForce=off  SenseConstraintForceX=off  SenseConstraintForceY=off  SenseConstraintForceZ=off  SenseConstraintTorque=off  SenseConstraintTorqueX=off  SenseConstraintTorqueY=off  SenseConstraintTorqueZ=off  SenseTotalForce=off  SenseTotalForceX=off  SenseTotalForceY=off  SenseTotalForceZ=off  SenseTotalTorque=off  SenseTotalTorqueX=off  SenseTotalTorqueY=off  SenseTotalTorqueZ=off  CompositeWrenchDir=FollowerOnBase  CompositeWrenchFrame=BaseFrame  EquilibriumPosition=0  EquilibriumPositionUnits=deg  SpringStiffness=0  SpringStiffnessUnits=N*m/deg  DampingCoefficient=0  DampingCoefficientUnits=N*m/(deg/s)  TorqueActuationMode=NoTorque  MotionActuationMode=ComputedMotion  SensePosition=on  SenseVelocity=off  SenseAcceleration=off  SenseTorqueForce=off  SenseLowerLimitTorqueForce=off  SenseUpperLimitTorqueForce=off  LowerLimitSpecify=off  LowerLimitBound=-90  LowerLimitBoundUnits=deg  LowerLimitStiffness=1e4  LowerLimitStiffnessUnits=N*m/deg  LowerLimitDamping=10  LowerLimitDampingUnits=N*m/(deg/s)  LowerLimitTransitionRegionWidth=0.1  LowerLimitTransitionRegionWidthUnits=deg  UpperLimitSpecify=off  UpperLimitBound=90  UpperLimitBoundUnits=deg  UpperLimitStiffness=1e4  UpperLimitStiffnessUnits=N*m/deg  UpperLimitDamping=10  UpperLimitDampingUnits=N*m/(deg/s)  UpperLimitTransitionRegionWidth=0.1  UpperLimitTransitionRegionWidthUnits=deg  PositionTargetSpecify=on  PositionTargetPriority=High  PositionTargetValue=0  PositionTargetValueUnits=deg  VelocityTargetSpecify=off  VelocityTargetPriority=High  VelocityTargetValue=0  VelocityTargetValueUnits=deg/s
  UArm to CrankL : sm_lib/Joints/Revolute Joint  JointMode=Normal  SenseConstraintForce=off  SenseConstraintForceX=off  SenseConstraintForceY=off  SenseConstraintForceZ=off  SenseConstraintTorque=off  SenseConstraintTorqueX=off  SenseConstraintTorqueY=off  SenseConstraintTorqueZ=off  SenseTotalForce=off  SenseTotalForceX=off  SenseTotalForceY=off  SenseTotalForceZ=off  SenseTotalTorque=off  SenseTotalTorqueX=off  SenseTotalTorqueY=off  SenseTotalTorqueZ=off  CompositeWrenchDir=FollowerOnBase  CompositeWrenchFrame=BaseFrame  EquilibriumPosition=0  EquilibriumPositionUnits=deg  SpringStiffness=0  SpringStiffnessUnits=N*m/deg  DampingCoefficient=0  DampingCoefficientUnits=N*m/(deg/s)  TorqueActuationMode=NoTorque  MotionActuationMode=ComputedMotion  SensePosition=off  SenseVelocity=off  SenseAcceleration=off  SenseTorqueForce=off  SenseLowerLimitTorqueForce=off  SenseUpperLimitTorqueForce=off  LowerLimitSpecify=off  LowerLimitBound=-90  LowerLimitBoundUnits=deg  LowerLimitStiffness=1e4  LowerLimitStiffnessUnits=N*m/deg  LowerLimitDamping=10  LowerLimitDampingUnits=N*m/(deg/s)  LowerLimitTransitionRegionWidth=0.1  LowerLimitTransitionRegionWidthUnits=deg  UpperLimitSpecify=off  UpperLimitBound=90  UpperLimitBoundUnits=deg  UpperLimitStiffness=1e4  UpperLimitStiffnessUnits=N*m/deg  UpperLimitDamping=10  UpperLimitDampingUnits=N*m/(deg/s)  UpperLimitTransitionRegionWidth=0.1  UpperLimitTransitionRegionWidthUnits=deg  PositionTargetSpecify=off  PositionTargetPriority=Low  PositionTargetValue=-150  PositionTargetValueUnits=deg  VelocityTargetSpecify=off  VelocityTargetPriority=High  VelocityTargetValue=0  VelocityTargetValueUnits=deg/s
  UArm to CrankR : sm_lib/Joints/Revolute Joint  JointMode=Normal  SenseConstraintForce=off  SenseConstraintForceX=off  SenseConstraintForceY=off  SenseConstraintForceZ=off  SenseConstraintTorque=off  SenseConstraintTorqueX=off  SenseConstraintTorqueY=off  SenseConstraintTorqueZ=off  SenseTotalForce=off  SenseTotalForceX=off  SenseTotalForceY=off  SenseTotalForceZ=off  SenseTotalTorque=off  SenseTotalTorqueX=off  SenseTotalTorqueY=off  SenseTotalTorqueZ=off  CompositeWrenchDir=FollowerOnBase  CompositeWrenchFrame=BaseFrame  EquilibriumPosition=0  EquilibriumPositionUnits=deg  SpringStiffness=0  SpringStiffnessUnits=N*m/deg  DampingCoefficient=0  DampingCoefficientUnits=N*m/(deg/s)  TorqueActuationMode=NoTorque  MotionActuationMode=ComputedMotion  SensePosition=off  SenseVelocity=off  SenseAcceleration=off  SenseTorqueForce=off  SenseLowerLimitTorqueForce=off  SenseUpperLimitTorqueForce=off  LowerLimitSpecify=off  LowerLimitBound=-90  LowerLimitBoundUnits=deg  LowerLimitStiffness=1e4  LowerLimitStiffnessUnits=N*m/deg  LowerLimitDamping=10  LowerLimitDampingUnits=N*m/(deg/s)  LowerLimitTransitionRegionWidth=0.1  LowerLimitTransitionRegionWidthUnits=deg  UpperLimitSpecify=off  UpperLimitBound=90  UpperLimitBoundUnits=deg  UpperLimitStiffness=1e4  UpperLimitStiffnessUnits=N*m/deg  UpperLimitDamping=10  UpperLimitDampingUnits=N*m/(deg/s)  UpperLimitTransitionRegionWidth=0.1  UpperLimitTransitionRegionWidthUnits=deg  PositionTargetSpecify=off  PositionTargetPriority=High  PositionTargetValue=0  PositionTargetValueUnits=deg  VelocityTargetSpecify=off  VelocityTargetPriority=High  VelocityTargetValue=0  VelocityTargetValueUnits=deg/s
  UArm to TActuator : sm_lib/Joints/Revolute Joint  JointMode=Normal  SenseConstraintForce=off  SenseConstraintForceX=off  SenseConstraintForceY=off  SenseConstraintForceZ=off  SenseConstraintTorque=off  SenseConstraintTorqueX=off  SenseConstraintTorqueY=off  SenseConstraintTorqueZ=off  SenseTotalForce=off  SenseTotalForceX=off  SenseTotalForceY=off  SenseTotalForceZ=off  SenseTotalTorque=off  SenseTotalTorqueX=off  SenseTotalTorqueY=off  SenseTotalTorqueZ=off  CompositeWrenchDir=FollowerOnBase  CompositeWrenchFrame=BaseFrame  EquilibriumPosition=0  EquilibriumPositionUnits=deg  SpringStiffness=0  SpringStiffnessUnits=N*m/deg  DampingCoefficient=0  DampingCoefficientUnits=N*m/(deg/s)  TorqueActuationMode=NoTorque  MotionActuationMode=ComputedMotion  SensePosition=off  SenseVelocity=off  SenseAcceleration=off  SenseTorqueForce=off  SenseLowerLimitTorqueForce=off  SenseUpperLimitTorqueForce=off  LowerLimitSpecify=off  LowerLimitBound=-90  LowerLimitBoundUnits=deg  LowerLimitStiffness=1e4  LowerLimitStiffnessUnits=N*m/deg  LowerLimitDamping=10  LowerLimitDampingUnits=N*m/(deg/s)  LowerLimitTransitionRegionWidth=0.1  LowerLimitTransitionRegionWidthUnits=deg  UpperLimitSpecify=off  UpperLimitBound=90  UpperLimitBoundUnits=deg  UpperLimitStiffness=1e4  UpperLimitStiffnessUnits=N*m/deg  UpperLimitDamping=10  UpperLimitDampingUnits=N*m/(deg/s)  UpperLimitTransitionRegionWidth=0.1  UpperLimitTransitionRegionWidthUnits=deg  PositionTargetSpecify=on  PositionTargetPriority=Low  PositionTargetValue=-90  PositionTargetValueUnits=deg  VelocityTargetSpecify=off  VelocityTargetPriority=High  VelocityTargetValue=0  VelocityTargetValueUnits=deg/s
  Upper Arm : Subsystem
      mask Display: image('Backhoe_Arm_Upper_IMAGE.jpg');
  World Frame : sm_lib/Frames and Transforms/World Frame
  Meas : Outport  VectorParamsAs1DForOutWhenUnconnected=off
  wires:
  Cmd3/1 -> Tilt Actuator/1(Cmd)
  Cmd2/1 -> Reach Actuator/1(Cmd)
  Measured/1(Angles) -> Meas/1
  Cmd/1 -> Lift Actuator/1(Cmd)
  connections:
  Reach Actuator/RConn2 -- "Lower Arm "/RConn2
  Upper Arm/RConn3 -- UArm to Bucket/LConn1
  "Lower Arm "/RConn1 -- LArm to UArm/LConn1
  Mech Config/RConn1 -- Mounting Hub/LConn1 -- Solver Config/RConn1 -- World Frame/RConn1
  "Lower Arm "/LConn1 -- Hub to LArm/RConn1
  Lift Actuator/RConn1 -- "Lower Arm "/LConn2
  Mounting Hub/RConn1 -- Hub to LArm/LConn1
  LArm to UArm/RConn1 -- Upper Arm/LConn1
  Reach Actuator/RConn1 -- Upper Arm/LConn2
  UArm to CrankR/LConn1 -- Upper Arm/RConn2
  UArm to CrankL/LConn1 -- Upper Arm/RConn1
  Sensing LAM/LConn1 -- Hub to LArm/RConn2
  Sensing LAU/LConn1 -- LArm to UArm/RConn2
  Sensing AB/LConn1 -- UArm to Bucket/RConn2
  Tilt Actuator/RConn1 -- Bucket Assembly/RConn1
  UArm to CrankL/RConn1 -- Bucket Assembly/LConn1
  UArm to CrankR/RConn1 -- Bucket Assembly/LConn2
  Bucket Assembly/LConn3 -- UArm to Bucket/RConn1
  Mounting Hub/RConn2 -- Lift Actuator/RConn2
  UArm to TActuator/LConn1 -- Upper Arm/RConn4
  Tilt Actuator/RConn2 -- UArm to TActuator/RConn1
  Pressure Relief Valve/LConn1 -- Sensing PA2/RConn1 -- Lift Actuator/LConn2 -- Tilt Actuator/LConn2 -- Reach Actuator/LConn2
  Pressure Relief Valve/RConn1 -- Hydraulic Fluid/RConn1 -- Tilt Actuator/LConn1 -- Reach Actuator/LConn1 -- Lift Actuator/LConn1 -- Hydraulic Reference/LConn1 -- Fixed- Displacement Pump/RConn2
  Pump Speed/RConn1 -- Ideal Angular Velocity Source/RConn1
  Ideal Angular Velocity Source/LConn1 -- Fixed- Displacement Pump/LConn1
  Mechanical Rotational Reference/LConn1 -- Ideal Angular Velocity Source/RConn2
  Sensing PA2/LConn1 -- Fixed- Displacement Pump/RConn1

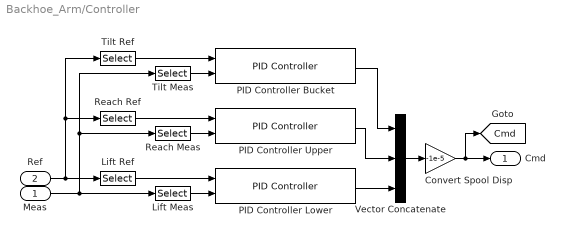
== system Backhoe_Arm/Controller ==
  Meas : Inport
  Ref : Inport  Port=2
  Convert Spool Disp : Gain  Gain=-1e-5
  Lift Meas : Selector  InputPortWidth=3  IndexOptions=Index vector (dialog)  Indices=3  OutputSizes=1
  Lift Ref : Selector  InputPortWidth=3  IndexOptions=Index vector (dialog)  Indices=3  OutputSizes=1
  PID Controller Bucket : Backhoe_Lib/PID Controller  upperLim=10  lowerLim=-120  Kp=10  Ki=0.01  Kd=0.01  N=100
  PID Controller Lower : Backhoe_Lib/PID Controller  upperLim=40  lowerLim=-70  Kp=30  Ki=0.002  Kd=0.002  N=100
  PID Controller Upper : Backhoe_Lib/PID Controller  upperLim=60  lowerLim=-20  Kp=24  Ki=0  Kd=0  N=100
  Reach Meas : Selector  InputPortWidth=3  IndexOptions=Index vector (dialog)  Indices=2  OutputSizes=1
  Reach Ref : Selector  InputPortWidth=3  IndexOptions=Index vector (dialog)  Indices=2  OutputSizes=1
  "Tilt Meas " : Selector  InputPortWidth=3  IndexOptions=Index vector (dialog)  Indices=1  OutputSizes=1
  Tilt Ref : Selector  InputPortWidth=3  IndexOptions=Index vector (dialog)  Indices=1  OutputSizes=1
  Vector Concatenate : Concatenate  NumInputs=3
  Cmd : Outport  VectorParamsAs1DForOutWhenUnconnected=off
  tag scope: Cmd=global
  wires:
  "Tilt Meas "/1 -> PID Controller Bucket/2
  Tilt Ref/1 -> PID Controller Bucket/1
  Reach Meas/1 -> PID Controller Upper/2
  Reach Ref/1 -> PID Controller Upper/1
  Lift Ref/1 -> PID Controller Lower/1
  Lift Meas/1 -> PID Controller Lower/2
  Meas/1 -> "Tilt Meas "/1, Reach Meas/1, Lift Meas/1
  Ref/1 -> Lift Ref/1, Tilt Ref/1, Reach Ref/1
  Vector Concatenate/1 -> Convert Spool Disp/1
  Convert Spool Disp/1 -> Cmd/1, [Cmd]
  PID Controller Upper/1 -> Vector Concatenate/2
  PID Controller Lower/1 -> Vector Concatenate/3
  PID Controller Bucket/1 -> Vector Concatenate/1

== system Backhoe_Arm/Routing ==
  Meas : Inport
  Demux : Demux  Outputs=3
  Demux1 : Demux  Outputs=3
  Mux : Mux  Inputs=2
  Mux1 : Mux  Inputs=2
  Mux2 : Mux  Inputs=2
  Bucket : Outport  VectorParamsAs1DForOutWhenUnconnected=off
  UArm : Outport  Port=2  VectorParamsAs1DForOutWhenUnconnected=off
  LArm : Outport  Port=3  VectorParamsAs1DForOutWhenUnconnected=off
  wires:
  Demux/3 -> Mux/1
  Demux/2 -> Mux1/1
  Demux1/1 -> Mux2/2
  Mux/1 -> LArm/1  "Lower Arm"
  Mux1/1 -> UArm/1  "Upper Arm"
  Demux/1 -> Mux2/1
  Demux1/3 -> Mux/2
  Demux1/2 -> Mux1/2
  Mux2/1 -> Bucket/1  "Bucket"
  [Ref] -> Demux1/1
  Meas/1 -> Demux/1

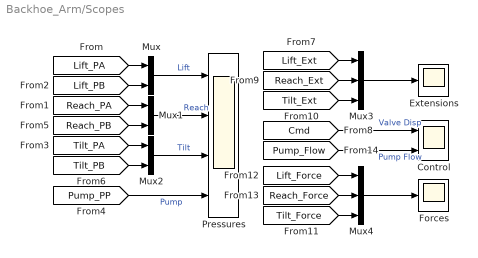
== system Backhoe_Arm/Scopes ==
  Control : Scope  NumInputPorts=2
  Extensions : Scope
  Forces : Scope
  Mux : Mux  Inputs=2
  Mux1 : Mux  Inputs=2
  Mux2 : Mux  Inputs=2
  Mux3 : Mux  Inputs=3
  Mux4 : Mux  Inputs=3
  Pressures : Scope  NumInputPorts=4
  wires:
  [Pump_PP] -> Pressures/4  "Pump"
  Mux/1 -> Pressures/1  "Lift"
  [Lift_PA] -> Mux/1
  [Lift_PB] -> Mux/2
  [Reach_PA] -> Mux1/1
  Mux1/1 -> Pressures/2  "Reach"
  [Reach_PB] -> Mux1/2
  [Tilt_PA] -> Mux2/1
  Mux2/1 -> Pressures/3  "Tilt"
  [Tilt_PB] -> Mux2/2
  [Lift_Ext] -> Mux3/1
  [Reach_Ext] -> Mux3/2
  [Tilt_Ext] -> Mux3/3
  Mux3/1 -> Extensions/1
  [Cmd] -> Control/1  "Valve Disp"
  [Lift_Force] -> Mux4/1
  [Reach_Force] -> Mux4/2
  [Tilt_Force] -> Mux4/3
  Mux4/1 -> Forces/1
  [Pump_Flow] -> Control/2  "Pump Flow"

== system Backhoe_Arm/Signal Builder ==
  Demux : Demux  Tag=STV Demux  Outputs=3
      settings: DisplayOption=none
  FromWs : FromWorkspace  Tag=STV FromWs  VariableName=tuvar  OutputAfterFinalValue=Holding final value
      SigBuilderData=|
      | common.afterFinalStr = 'Hold final value'
      | common.sampleTime = '0'
      | dataSet.timeRange = [0 60]
      | dataSet.name = 'Ref'
      | sbobj.Groups.Name = 'Ref'
      | sbobj.Groups.Signals(1).Name = 'Bucket Angle'
      | sbobj.Groups.Signals(1).XData = [0 7 11 24 28.5 40 43 51.5 53.5 60]
      | sbobj.Groups.Signals(1).YData = [0 0 -90 -90 0 0 -110 -110 0 0]
      | sbobj.Groups.Signals(2).Name = 'Upper Angle'
      | sbobj.Groups.Signals(2).XData = [0 12.5 25 30 32.5 54 60]
      | sbobj.Groups.Signals(2).YData = [50 50 -20 -20 40 55 55]
      | sbobj.Groups.Signals(3).Name = 'Lower Angle'
      | sbobj.Groups.Signals(3).XData = [0 15 27.5 30 40 60]
      | sbobj.Groups.Signals(3).YData = [-60 -60 -30 -30 -60 -60]
      | sbobj.Groups.TimeRange = [0 60]
  Bucket Angle : Outport  Tag=STV Outport  VectorParamsAs1DForOutWhenUnconnected=off
  Upper Angle : Outport  Tag=STV Outport  Port=2  VectorParamsAs1DForOutWhenUnconnected=off
  Lower Angle : Outport  Tag=STV Outport  Port=3  VectorParamsAs1DForOutWhenUnconnected=off
  wires:
  Demux/3 -> Lower Angle/1
  Demux/2 -> Upper Angle/1
  FromWs/1 -> Demux/1
  Demux/1 -> Bucket Angle/1

== system Backhoe_Arm/xPC Scope ==
  In1 : Inport
  "Scope (xPC) " : slrtlib/Displays and Logging/Scope   scopeno=2  scopetype=Target  autostart=on  viewmode=Graphical redraw  formatstr='%15.6f'  grid=on  ylimits=[-100, 0]  nosamples=2500  noprepostsamples=0  interleave=1  triggermode=FreeRun  triggersignal=1  trigsignalfromport=off  triggerlevel=0.0  triggerslope=Either  triggerscope=1  triggersample=0  filename=data.dat  mode=Lazy  writesize=512  autorestart=off  dynamicfilemode=off  maxwritefilesize=512*1024^2
  wires:
  In1/1 -> "Scope (xPC) "/1

== system Backhoe_Arm/Arm/Bucket Assembly ==
  Bucket : Subsystem  mask(Bucket){plateSide=1.2, plateFilletR=0.2, plateDist=1.2, plateWidth=0.2, plateHoleR=0.075, bucketHeight=2, bucketLength=2, bucketThickness=0.05, bucketUpper=1.3, bucketLower=2, chordAngle=pi/6, toothLength=0.25, toothWidth=0.2, toothTip=0.025, circlePoints=45, bucketColor=yellow, bracketColor=yellow, rho=rhoSteel}
      mask prompts: plateSide "Wplate [m]"; plateFilletR "Rfillet [m]"; plateDist "Dplate [m]"; plateWidth "Tplate [m]"; plateHoleR "Rpin [m]"; bucketHeight "Hbucket [m]"; bucketLength "Wbucket [m]"; bucketThickness "Tbucket [m]"; bucketUpper "Wupper [m]"; bucketLower "Wlower [m]"; chordAngle "alpha [radians]"; toothLength "Ltooth [m]"; toothWidth "Wtooth [m]"; toothTip "Ttooth [m]"; circlePoints "Circle Mesh Resolution"; bucketColor "Bucket Color"; bracketColor "Bracket Color"; rho "Density [kg/m^3]"
      mask help:
      | Consists of the backhoe bucket assembly with attachment frame.
      |
      | Attachment points are:
      | CA: Center point of the Crank Arm link pin.
      | UA: Center Point of the Upper Arm link pin.
      | Both points are configured for Revolute joints.
      |
      | Click on Help to view a schematic of the bucket, its configurable dimension parameters and attachment points (in red).
      mask init:
      | bucketRadius = bucketHeight/(2*cos(chordAngle));
      | 
      | % Bucket Back
      | bucketBack = [];
      | % Outer wall
      | for i = 0:circlePoints;
      |    angle = (-pi/2+chordAngle) + (pi - 2*chordAngle)*(i/circlePoints);
      |    bucketBack = [bucketBack; ...
      |        (bucketRadius*cos(angle)-bucketRadius*sin(chordAngle)) ...
      |         bucketRadius*sin(angle)];
      | end
      | 
      | % Inner Wall
      | beta = acos( ( (bucketRadius*cos(chordAngle) - bucketThickness/cos(chordAngle)) ...
      |                    /(bucketRadius-bucketThickness)) );
      | for i = 0:circlePoints;
      |    angle = (pi/2 - beta) - (pi-2*beta)*(i/circlePoints);
      |    bucketBack = [bucketBack; ...
      |        ((bucketRadius-bucketThickness)*cos(angle)-bucketRadius*sin(chordAngle)) ... 
      |        (bucketRadius-bucketThickness)*sin(angle)];
      | end
      | 
      | bucketBack = [bucketBack; ...
      |               -bucketLower -(bucketHeight/2-bucketThickness);...
      |               -bucketLower -bucketHeight/2];
      |           
      | % Uncomment below to plot the cross-sections. 
      | % close all
      | % figure
      | % plot(bucketBack(:,1),bucketBack(:,2));
      mask Help: web('Backhoe_Bucket.html');
      mask DialogControl ParameterTabVar0 Prompt: Attachment Frame
      mask DialogControl ParameterTabVar01 Prompt: Bucket
      mask DialogControl ParameterTabVar012 Prompt: Material Properties
      mask Display:
      | image('Backhoe_Bucket_IMAGE.png');
      | port_label('rconn',1,'CA');
      | port_label('rconn',2,'UA');
  Crank Assembly : Subsystem  mask(Crank Assembly){LC1=1.5, WC1=0.4, TC1=0.2, DH1=1.1, RH1=0.075, LC2=1.75, WC2=0.4, TC2=0.15, DH2=1.35, RH2=0.075, DC2=0.7, Wbar=0.8, Lpin=1.3, Rpin=0.075, circlePoints=25, color1=orange, color2=darkOrange, rho1=rhoSteel, rho2=rhoSteel}
      mask prompts: LC1 "LC1 [m]"; WC1 "WC1 [m]"; TC1 "TC1 [m]"; DH1 "DH1 [m]"; RH1 "RH1 [m]"; LC2 "LC2 [m]"; WC2 "WC2 [m]"; TC2 "TC2 [m]"; DH2 "DH2 [m]"; RH2 "RH2 [m]"; DC2 "DC2 [m]"; Wbar "Upper Arm Width, Wbar [m]"; Lpin "Lpin [m]"; Rpin "Rpin [m]"; circlePoints "Circle Mesh Resolution"; color1 "Color"; color2 "Color"; rho1 "Density [kg/m^3]"; rho2 "Density [kg/m^3]"
      mask help:
      | Consists of the backhoe crank assembly that connects the upper arm and the bucket. Crank 1 attaches to either side of the upper arm linkage, and Crank 2 connects Crank 1 and the Bucket.
      |
      | Attachment points are:
      | AL: Arm attachment (Left).
      | AR: Arm attachment (Right).
      | B: Bucket attachment.
      | P: Piston attachment.
      | All attachment points are configured for Revolute joints.
      |
      | Click on Help to view a schematic of the crank assembly, its configurable dimension parameters and attachment points (in red).
      mask Help: web('Backhoe_Crank.html');
      mask DialogControl ParameterTabVar0 Prompt: Crank 1
      mask DialogControl ParameterTabVar01 Prompt: Crank 2
      mask DialogControl ParameterTabVar012 Prompt: Other
      mask Display:
      | image('Backhoe_Crankassembly_IMAGE.png');
      | port_label('rconn',1,'B');
      | port_label('rconn',2,'P');
      | port_label('lconn',1,'AL');
      | port_label('lconn',2,'AR');
  Crank to Bucket : sm_lib/Joints/Revolute Joint  JointMode=Normal  SenseConstraintForce=off  SenseConstraintForceX=off  SenseConstraintForceY=off  SenseConstraintForceZ=off  SenseConstraintTorque=off  SenseConstraintTorqueX=off  SenseConstraintTorqueY=off  SenseConstraintTorqueZ=off  SenseTotalForce=off  SenseTotalForceX=off  SenseTotalForceY=off  SenseTotalForceZ=off  SenseTotalTorque=off  SenseTotalTorqueX=off  SenseTotalTorqueY=off  SenseTotalTorqueZ=off  CompositeWrenchDir=FollowerOnBase  CompositeWrenchFrame=BaseFrame  EquilibriumPosition=0  EquilibriumPositionUnits=deg  SpringStiffness=0  SpringStiffnessUnits=N*m/deg  DampingCoefficient=0  DampingCoefficientUnits=N*m/(deg/s)  TorqueActuationMode=NoTorque  MotionActuationMode=ComputedMotion  SensePosition=off  SenseVelocity=off  SenseAcceleration=off  SenseTorqueForce=off  SenseLowerLimitTorqueForce=off  SenseUpperLimitTorqueForce=off  LowerLimitSpecify=off  LowerLimitBound=-90  LowerLimitBoundUnits=deg  LowerLimitStiffness=1e4  LowerLimitStiffnessUnits=N*m/deg  LowerLimitDamping=10  LowerLimitDampingUnits=N*m/(deg/s)  LowerLimitTransitionRegionWidth=0.1  LowerLimitTransitionRegionWidthUnits=deg  UpperLimitSpecify=off  UpperLimitBound=90  UpperLimitBoundUnits=deg  UpperLimitStiffness=1e4  UpperLimitStiffnessUnits=N*m/deg  UpperLimitDamping=10  UpperLimitDampingUnits=N*m/(deg/s)  UpperLimitTransitionRegionWidth=0.1  UpperLimitTransitionRegionWidthUnits=deg  PositionTargetSpecify=off  PositionTargetPriority=Low  PositionTargetValue=0  PositionTargetValueUnits=deg  VelocityTargetSpecify=off  VelocityTargetPriority=High  VelocityTargetValue=0  VelocityTargetValueUnits=deg/s
  TAct : PMIOPort  Side=Right
  UAL : PMIOPort  Port=2  Side=Left
  UAR : PMIOPort  Port=3  Side=Left
  UA : PMIOPort  Port=4  Side=Left
  connections:
  Bucket/RConn1 -- Crank to Bucket/RConn1
  Crank Assembly/RConn2 -- Crank to Bucket/LConn1
  Bucket/RConn2 -- UA/RConn1
  UAL/RConn1 -- Crank Assembly/LConn1
  UAR/RConn1 -- Crank Assembly/LConn2
  TAct/RConn1 -- Crank Assembly/RConn1
